simulink model "pil_left"  (R2021a)
settings: Solver=FixedStepAuto  StartTime=0.0  StopTime=inf  RelTol=1e-3  EnableMultiTasking=on
libraries: pil_lib x1
settings Model: Creator=Abbas  LastModifiedBy=Abbas
settings OptimizationCC: EnhancedBackFolding=on  PassReuseOutputArgsAs=Individual arguments  ZeroExternalMemoryAtStartup=off  ZeroInternalMemoryAtStartup=off  MaxStackSize=64  OptimizeBlockOrder=speed  DifferentSizesBufferReuse=on  OptimizationCustomize=off  EfficientTunableParamExpr=on
settings DebuggingCC: ParameterTunabilityLossMsg=error
settings HardwareCC: ProdBitPerInt=16  ProdBitPerPointer=16  ProdBitPerSizeT=16  ProdBitPerPtrDiffT=16  ProdLargestAtomicFloat=None  ProdWordSize=8  ProdHWDeviceType=Atmel->AVR
settings SFSimCC: MATLABDynamicMemAlloc=off
settings RTWCC: SystemTargetFile=ert.tlc  HardwareBoard=Arduino Uno  TemplateMakefile=ert_default_tmf  Toolchain=Arduino AVR  BuildConfiguration=Faster Runs  PortableWordSizes=on  CreateSILPILBlock=PIL
settings CodeAppCC: ForceParamTrailComments=on  IgnoreCustomStorageClasses=off  OperatorAnnotations=on  SimulinkDataObjDesc=on  SFDataObjDesc=on  InsertBlockDesc=on
settings ERTTargetCC: SupportContinuousTime=on  SupportVariableSizeSignals=on  ExtModeStaticAllocSize=250

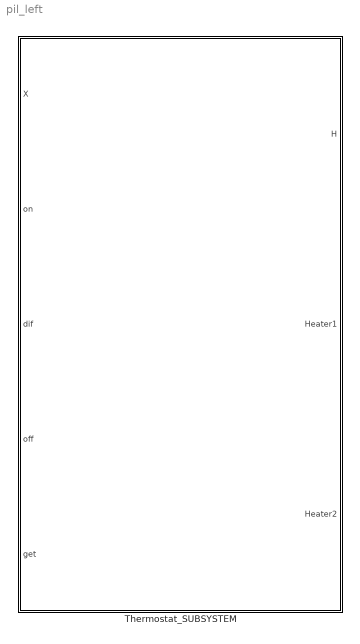
== system pil_left ==
  Thermostat_SUBSYSTEM : Subsystem  DialogController=pil_create_dialog  LoadFcn=|
      | try
      |    if ~strcmp(rtw.pil.getPILVersion, '9.10 (R2021a)_15')
      |       set_param(gcb, 'DialogController', '');
      |       set_param(gcb, 'DialogControllerArgs', '');
      |    end
      | catch e
      |       set_param(gcb, 'DialogController', '');
      |       set_param(gcb, 'DialogControllerArgs', '');
      | end
      mask help: PIL:pil:XILBlockMaskDesc
      mask Display: disp('PIL');

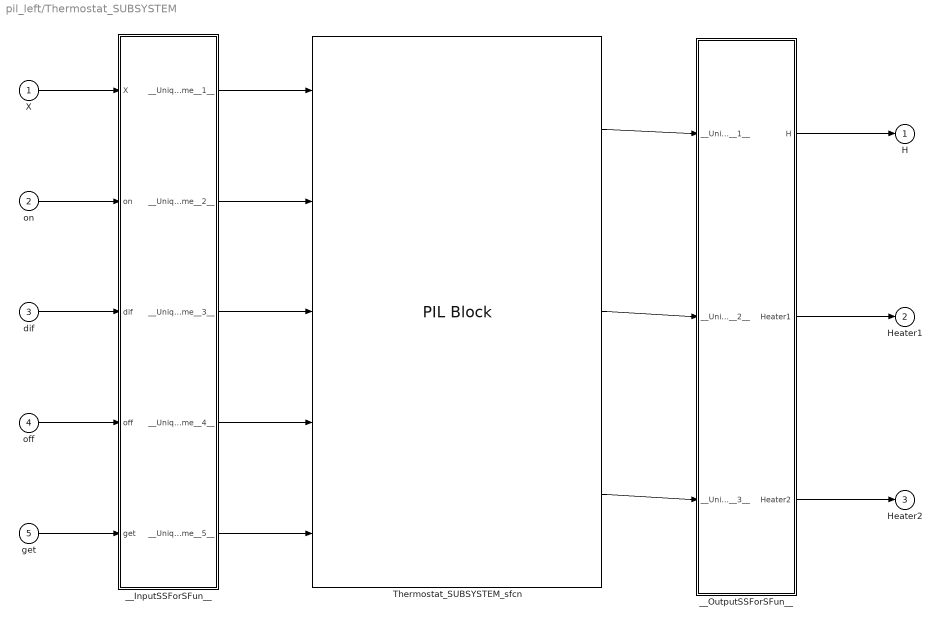
== system pil_left/Thermostat_SUBSYSTEM ==
  X : Inport
  on : Inport  Port=2
  dif : Inport  Port=3
  off : Inport  Port=4
  get : Inport  Port=5
  Thermostat_SUBSYSTEM_sfcn : pil_lib/PIL Block  SimulationMode=PIL  IsTopModelPIL=off  CodeDir=D:\desktop\embedded\HW\embedded_system\final_project\last\Thermostat_SUBSYSTEM_ert_rtw  AnchorDir=D:\desktop\embedded\HW\embedded_system\final_project\last  ConfigName=Arduino Board  XrelIsTopModelCode=on  XrelIsReusable=off  XrelDWorkNames={}  XrelDWorkTypes={}  XrelModelArgVals={}  XrelOrderedParamNames={}
      settings: SourceProductBaseCode=RT
  __InputSSForSFun__ : Subsystem
  __OutputSSForSFun__ : Subsystem
  H : Outport
  Heater1 : Outport  Port=2
  Heater2 : Outport  Port=3
  wires:
  X/1 -> __InputSSForSFun__/1(X)
  on/1 -> __InputSSForSFun__/2(on)
  dif/1 -> __InputSSForSFun__/3(dif)
  off/1 -> __InputSSForSFun__/4(off)
  get/1 -> __InputSSForSFun__/5(get)
  __InputSSForSFun__/1(__UniqueOutportName__1__) -> Thermostat_SUBSYSTEM_sfcn/1
  __InputSSForSFun__/2(__UniqueOutportName__2__) -> Thermostat_SUBSYSTEM_sfcn/2
  __InputSSForSFun__/3(__UniqueOutportName__3__) -> Thermostat_SUBSYSTEM_sfcn/3
  __InputSSForSFun__/4(__UniqueOutportName__4__) -> Thermostat_SUBSYSTEM_sfcn/4
  __InputSSForSFun__/5(__UniqueOutportName__5__) -> Thermostat_SUBSYSTEM_sfcn/5
  Thermostat_SUBSYSTEM_sfcn/1 -> __OutputSSForSFun__/1(__UniqueInportName__1__)
  Thermostat_SUBSYSTEM_sfcn/2 -> __OutputSSForSFun__/2(__UniqueInportName__2__)
  Thermostat_SUBSYSTEM_sfcn/3 -> __OutputSSForSFun__/3(__UniqueInportName__3__)
  __OutputSSForSFun__/1(H) -> H/1
  __OutputSSForSFun__/2(Heater1) -> Heater1/1
  __OutputSSForSFun__/3(Heater2) -> Heater2/1

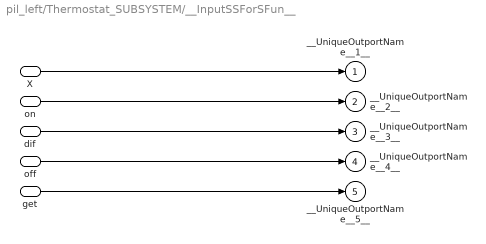
== system pil_left/Thermostat_SUBSYSTEM/__InputSSForSFun__ ==
  X : Inport
  on : Inport  Port=2
  dif : Inport  Port=3
  off : Inport  Port=4
  get : Inport  Port=5
  __UniqueOutportName__1__ : Outport
  __UniqueOutportName__2__ : Outport  Port=2
  __UniqueOutportName__3__ : Outport  Port=3
  __UniqueOutportName__4__ : Outport  Port=4
  __UniqueOutportName__5__ : Outport  Port=5
  wires:
  X/1 -> __UniqueOutportName__1__/1
  on/1 -> __UniqueOutportName__2__/1
  dif/1 -> __UniqueOutportName__3__/1
  off/1 -> __UniqueOutportName__4__/1
  get/1 -> __UniqueOutportName__5__/1

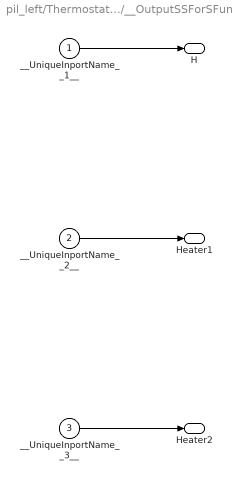
== system pil_left/Thermostat_SUBSYSTEM/__OutputSSForSFun__ ==
  __UniqueInportName__1__ : Inport
  __UniqueInportName__2__ : Inport  Port=2
  __UniqueInportName__3__ : Inport  Port=3
  H : Outport
  Heater1 : Outport  Port=2
  Heater2 : Outport  Port=3
  wires:
  __UniqueInportName__1__/1 -> H/1
  __UniqueInportName__2__/1 -> Heater1/1
  __UniqueInportName__3__/1 -> Heater2/1
